simulink model "simulink_model"  (R2020b)
settings: Solver=VariableStepAuto  StartTime=0.0  StopTime=10  MaxStep=1e-3  RelTol=1e-5  AbsTol=1e-5
InitFcn:
  | % Init Walking SLIP
  | m = 80;
  | g = 9.81;
  | kk = 10000;
  | l0 = 1;
  | aTD = 68*pi/180;
  | E = 810;
  | x0 = 0;
  | y0 = 0.97;
  | dx0 = 1.05;
  | dy0 = 0;
  | yTD = l0*sin(aTD);
settings Model: Creator=ASUS  LastModifiedBy=edizferit
settings DataIOCC: ReturnWorkspaceOutputs=off

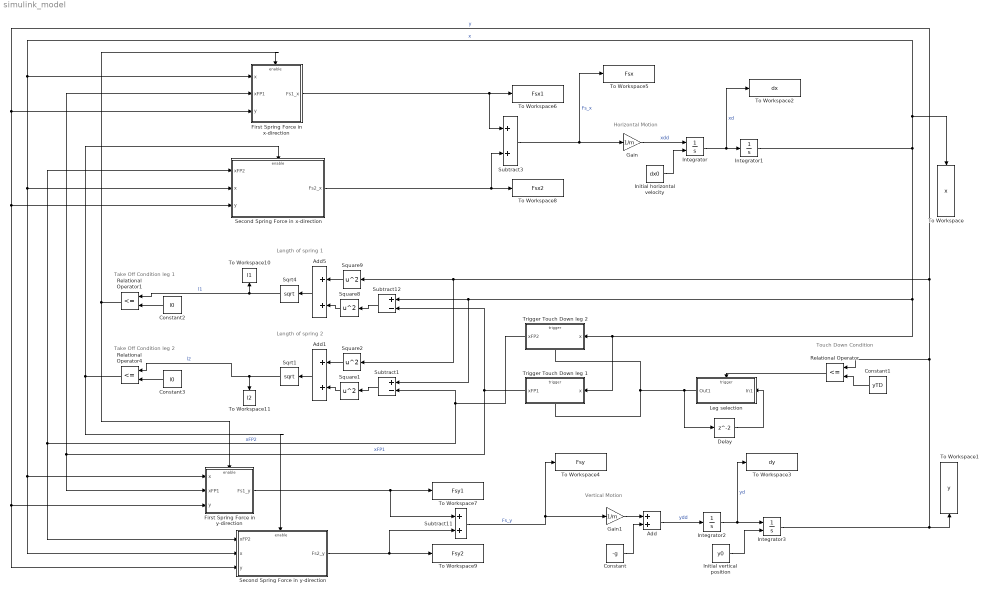
== system simulink_model ==
  note: Touch Down Condition
  note: Take Off Condition leg 1
  note: Vertical Motion
  note: Horizontal Motion
  note: Length of spring 1
  note: Length of spring 2
  note: Take Off Condition leg 2
  Add : Sum
  Add1 : Sum
  Add5 : Sum
  Constant : Constant  Value=-g
  Constant1 : Constant  Value=yTD
  Constant2 : Constant  Value=l0
  Constant3 : Constant  Value=l0
  Delay : Delay
  First Spring Force in x-direction : Subsystem
  First Spring Force in y-direction : Subsystem
  Gain : Gain  Gain=1/m
  Gain1 : Gain  Gain=1/m
  Initial horizontal velocity : Constant  InitFcn=|  Value=dx0
      | %% Init Running SLIP
      | m = 80;
      | g = 9.81;
      | k = 10;
      | l0 = 1;
      | aTD = 68*pi/180;
      | E = 810;
      | x0 = 0;
      | y0 = 0.97;
      | dx0 = 1.05;
      | dy0 = 0;
      | yTD = l0*sin(aTD);
  Initial vertical position : Constant  Value=y0
  Integrator : Integrator  InitialConditionSource=external
  Integrator1 : Integrator
  Integrator2 : Integrator
  Integrator3 : Integrator  InitialConditionSource=external
  "Leg selection " : Subsystem  TreatAsAtomicUnit=on
  Relational Operator : RelationalOperator  Operator=<=  OutDataTypeStr=boolean  RndMeth=Simplest
  Relational Operator1 : RelationalOperator  Operator=<=  OutDataTypeStr=boolean  RndMeth=Simplest
  Relational Operator4 : RelationalOperator  Operator=<=  OutDataTypeStr=boolean  RndMeth=Simplest
  Second Spring Force in x-direction : Subsystem
  Second Spring Force in y-direction : Subsystem
  Sqrt1 : Sqrt  SaturateOnIntegerOverflow=on
  Sqrt4 : Sqrt  SaturateOnIntegerOverflow=on
  Square{1..2,8..9} (4 alike) : Math  Operator=square  SaturateOnIntegerOverflow=on
  Subtract1 : Sum  Inputs=+-
  Subtract11 : Sum
  Subtract12 : Sum  Inputs=+-
  Subtract3 : Sum
  To Workspace : ToWorkspace  VariableName=x  SaveFormat=Timeseries  SampleTime=-1
  To Workspace1 : ToWorkspace  VariableName=y  SaveFormat=Timeseries  SampleTime=-1
  To Workspace10 : ToWorkspace  VariableName=l1  SaveFormat=Timeseries  SampleTime=-1
  To Workspace11 : ToWorkspace  VariableName=l2  SaveFormat=Timeseries  SampleTime=-1
  To Workspace2 : ToWorkspace  VariableName=dx  SaveFormat=Timeseries  SampleTime=-1
  To Workspace3 : ToWorkspace  VariableName=dy  SaveFormat=Timeseries  SampleTime=-1
  To Workspace4 : ToWorkspace  VariableName=Fsy  SaveFormat=Timeseries  SampleTime=-1
  To Workspace5 : ToWorkspace  VariableName=Fsx  SaveFormat=Timeseries  SampleTime=-1
  To Workspace6 : ToWorkspace  VariableName=Fsx1  SaveFormat=Timeseries  SampleTime=-1
  To Workspace7 : ToWorkspace  VariableName=Fsy1  SaveFormat=Timeseries  SampleTime=-1
  To Workspace8 : ToWorkspace  VariableName=Fsx2  SaveFormat=Timeseries  SampleTime=-1
  To Workspace9 : ToWorkspace  VariableName=Fsy2  SaveFormat=Timeseries  SampleTime=-1
  Trigger Touch Down leg 1 : Subsystem  TreatAsAtomicUnit=on
  Trigger Touch Down leg 2 : Subsystem  TreatAsAtomicUnit=on
  wires:
  Gain/1 -> Integrator/1  "xdd"
  Integrator/1 -> To Workspace2/1, Integrator1/1  "xd"
  Initial horizontal velocity/1 -> Integrator/2
  Initial vertical position/1 -> Integrator3/2
  Add/1 -> Integrator2/1  "ydd"
  Gain1/1 -> Add/1
  Constant/1 -> Add/2
  Constant1/1 -> Relational Operator/2
  Constant2/1 -> Relational Operator1/2
  Sqrt4/1 -> Relational Operator1/1, To Workspace10/1  "l1"
  Integrator3/1 -> Second Spring Force in y-direction/3(y), First Spring Force in y-direction/3(y), Second Spring Force in x-direction/3(y), First Spring Force in x-direction/3(y), Square2/1, Square9/1, Relational Operator/1, To Workspace1/1  "y"
  Subtract12/1 -> Square8/1
  Add5/1 -> Sqrt4/1
  Square9/1 -> Add5/1
  Square8/1 -> Add5/2
  Trigger Touch Down leg 2/1(xFP2) -> Second Spring Force in x-direction/1(xFP2), Second Spring Force in y-direction/1(xFP2), Subtract1/2  "xFP2"
  Trigger Touch Down leg 1/1(xFP1) -> First Spring Force in x-direction/2(xFP1), First Spring Force in y-direction/2(xFP1), Subtract12/2  "xFP1"
  Second Spring Force in y-direction/1(Fs2_y) -> To Workspace9/1, Subtract11/2
  First Spring Force in y-direction/1(Fs1_y) -> To Workspace7/1, Subtract11/1
  First Spring Force in x-direction/1(Fs1_x) -> To Workspace6/1, Subtract3/1
  Second Spring Force in x-direction/1(Fs2_x) -> To Workspace8/1, Subtract3/2
  Relational Operator/1 -> "Leg selection "/Trigger
  "Leg selection "/1(Out1) -> Delay/1, Trigger Touch Down leg 2/Trigger, Trigger Touch Down leg 1/Trigger
  Delay/1 -> "Leg selection "/1(In1)
  Square1/1 -> Add1/2
  Square2/1 -> Add1/1
  Add1/1 -> Sqrt1/1
  Subtract1/1 -> Square1/1
  Constant3/1 -> Relational Operator4/2
  Sqrt1/1 -> Relational Operator4/1, To Workspace11/1  "l2"
  Relational Operator1/1 -> First Spring Force in x-direction/Enable, First Spring Force in y-direction/Enable
  Relational Operator4/1 -> Second Spring Force in x-direction/Enable, Second Spring Force in y-direction/Enable
  Integrator2/1 -> To Workspace3/1, Integrator3/1  "yd"
  Subtract11/1 -> To Workspace4/1, Gain1/1  "Fs_y"
  Integrator1/1 -> To Workspace/1, Second Spring Force in y-direction/2(x), First Spring Force in y-direction/1(x), Second Spring Force in x-direction/2(x), First Spring Force in x-direction/1(x), Trigger Touch Down leg 1/1(x), Trigger Touch Down leg 2/1(x), Subtract12/1, Subtract1/1  "x"
  Subtract3/1 -> To Workspace5/1, Gain/1  "Fs_x"

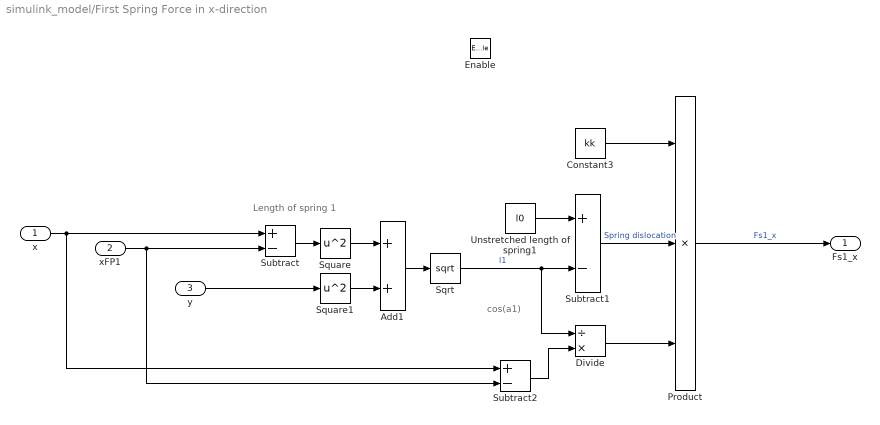
== system simulink_model/First Spring Force in x-direction ==
  note: cos(a1)
  note: Length of spring 1
  x : Inport
  xFP1 : Inport  Port=2
  y : Inport  Port=3
  Enable : EnablePort  StatesWhenEnabling=reset
  Add1 : Sum
  Constant3 : Constant  Value=kk
  Divide : Product  Inputs=/*
  Product : Product  Inputs=3
  Sqrt : Sqrt  SaturateOnIntegerOverflow=on
  Square : Math  Operator=square  SaturateOnIntegerOverflow=on
  Square1 : Math  Operator=square  SaturateOnIntegerOverflow=on
  Subtract : Sum  Inputs=+-
  Subtract1 : Sum  Inputs=+-
  Subtract2 : Sum  Inputs=+-
  Unstretched length of spring1 : Constant  Value=l0
  Fs1_x : Outport
  wires:
  Sqrt/1 -> Divide/1, Subtract1/2  "l1"
  Add1/1 -> Sqrt/1
  Subtract/1 -> Square/1
  Constant3/1 -> Product/1
  Subtract1/1 -> Product/2  "Spring dislocation"
  Unstretched length of spring1/1 -> Subtract1/1
  Square1/1 -> Add1/2
  Divide/1 -> Product/3
  Subtract2/1 -> Divide/2
  Square/1 -> Add1/1
  xFP1/1 -> Subtract2/2, Subtract/2
  x/1 -> Subtract2/1, Subtract/1
  Product/1 -> Fs1_x/1  "Fs1_x"
  y/1 -> Square1/1

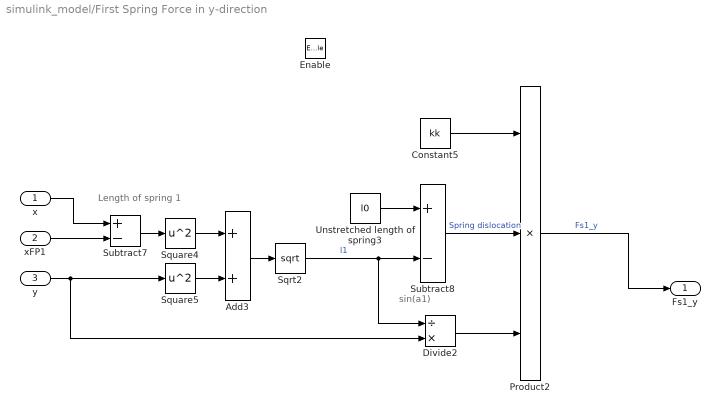
== system simulink_model/First Spring Force in y-direction ==
  note: sin(a1)
  note: Length of spring 1
  x : Inport
  xFP1 : Inport  Port=2
  y : Inport  Port=3
  Enable : EnablePort  StatesWhenEnabling=reset
  Add3 : Sum
  Constant5 : Constant  Value=kk
  Divide2 : Product  Inputs=/*
  Product2 : Product  Inputs=3
  Sqrt2 : Sqrt  SaturateOnIntegerOverflow=on
  Square4 : Math  Operator=square  SaturateOnIntegerOverflow=on
  Square5 : Math  Operator=square  SaturateOnIntegerOverflow=on
  Subtract7 : Sum  Inputs=+-
  Subtract8 : Sum  Inputs=+-
  Unstretched length of spring3 : Constant  Value=l0
  Fs1_y : Outport
  wires:
  Subtract8/1 -> Product2/2  "Spring dislocation"
  Divide2/1 -> Product2/3
  Unstretched length of spring3/1 -> Subtract8/1
  Subtract7/1 -> Square4/1
  Add3/1 -> Sqrt2/1
  Square5/1 -> Add3/2
  Sqrt2/1 -> Divide2/1, Subtract8/2  "l1"
  Square4/1 -> Add3/1
  x/1 -> Subtract7/1
  Constant5/1 -> Product2/1
  y/1 -> Divide2/2, Square5/1
  xFP1/1 -> Subtract7/2
  Product2/1 -> Fs1_y/1  "Fs1_y"

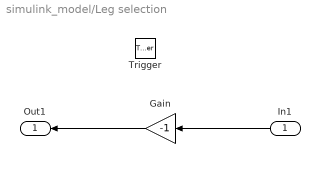
== system simulink_model/Leg selection  ==
  In1 : Inport
  Trigger : TriggerPort  VariantControl=Variant
  Gain : Gain  Gain=-1
  Out1 : Outport  InitialOutput=[1]
  wires:
  In1/1 -> Gain/1
  Gain/1 -> Out1/1

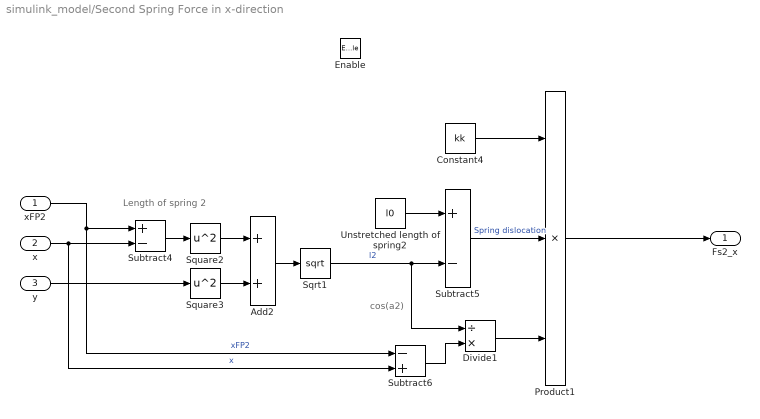
== system simulink_model/Second Spring Force in x-direction ==
  note: cos(a2)
  note: Length of spring 2
  xFP2 : Inport
  x : Inport  Port=2
  y : Inport  Port=3
  Enable : EnablePort  StatesWhenEnabling=reset
  Add2 : Sum
  Constant4 : Constant  Value=kk
  Divide1 : Product  Inputs=/*
  Product1 : Product  Inputs=3
  Sqrt1 : Sqrt  SaturateOnIntegerOverflow=on
  Square2 : Math  Operator=square  SaturateOnIntegerOverflow=on
  Square3 : Math  Operator=square  SaturateOnIntegerOverflow=on
  Subtract4 : Sum  Inputs=+-
  Subtract5 : Sum  Inputs=+-
  Subtract6 : Sum  Inputs=-+
  Unstretched length of spring2 : Constant  Value=l0
  Fs2_x : Outport  OutputWhenDisabled=reset  InitialOutput=[0]
  wires:
  Subtract4/1 -> Square2/1
  Sqrt1/1 -> Divide1/1, Subtract5/2  "l2"
  Subtract6/1 -> Divide1/2
  Square3/1 -> Add2/2
  Square2/1 -> Add2/1
  xFP2/1 -> Subtract6/1, Subtract4/1  "xFP2"
  x/1 -> Subtract6/2, Subtract4/2  "x"
  Constant4/1 -> Product1/1
  Divide1/1 -> Product1/3
  Unstretched length of spring2/1 -> Subtract5/1
  Add2/1 -> Sqrt1/1
  Subtract5/1 -> Product1/2  "Spring dislocation"
  Product1/1 -> Fs2_x/1
  y/1 -> Square3/1

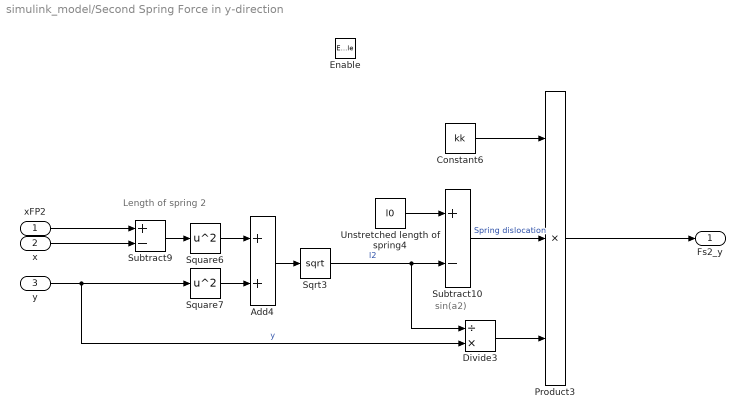
== system simulink_model/Second Spring Force in y-direction ==
  note: sin(a2)
  note: Length of spring 2
  xFP2 : Inport
  x : Inport  Port=2
  y : Inport  Port=3
  Enable : EnablePort  StatesWhenEnabling=reset
  Add4 : Sum
  Constant6 : Constant  Value=kk
  Divide3 : Product  Inputs=/*
  Product3 : Product  Inputs=3
  Sqrt3 : Sqrt  SaturateOnIntegerOverflow=on
  Square6 : Math  Operator=square  SaturateOnIntegerOverflow=on
  Square7 : Math  Operator=square  SaturateOnIntegerOverflow=on
  Subtract10 : Sum  Inputs=+-
  Subtract9 : Sum  Inputs=+-
  Unstretched length of spring4 : Constant  Value=l0
  Fs2_y : Outport  OutputWhenDisabled=reset  InitialOutput=[0]
  wires:
  Unstretched length of spring4/1 -> Subtract10/1
  Constant6/1 -> Product3/1
  Add4/1 -> Sqrt3/1
  Subtract9/1 -> Square6/1
  Square7/1 -> Add4/2
  Square6/1 -> Add4/1
  Sqrt3/1 -> Divide3/1, Subtract10/2  "l2"
  Divide3/1 -> Product3/3
  Subtract10/1 -> Product3/2  "Spring dislocation"
  x/1 -> Subtract9/2
  y/1 -> Divide3/2, Square7/1  "y"
  xFP2/1 -> Subtract9/1
  Product3/1 -> Fs2_y/1

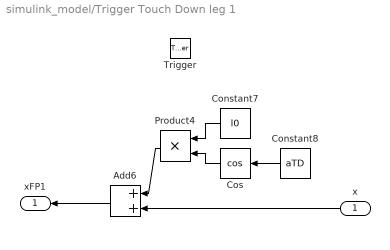
== system simulink_model/Trigger Touch Down leg 1 ==
  x : Inport
  Trigger : TriggerPort  VariantControl=Variant
  Add6 : Sum
  Constant7 : Constant  Value=l0
  Constant8 : Constant  Value=aTD
  Cos : Trigonometry  Operator=cos
  Product4 : Product
  xFP1 : Outport  InitialOutput=[0]
  wires:
  x/1 -> Add6/2
  Constant8/1 -> Cos/1
  Add6/1 -> xFP1/1
  Constant7/1 -> Product4/1
  Product4/1 -> Add6/1
  Cos/1 -> Product4/2

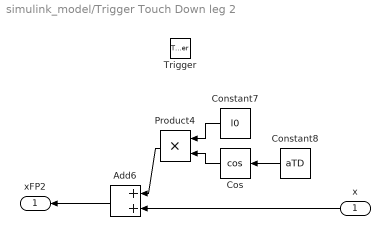
== system simulink_model/Trigger Touch Down leg 2 ==
  x : Inport
  Trigger : TriggerPort  TriggerType=falling  VariantControl=Variant
  Add6 : Sum
  Constant7 : Constant  Value=l0
  Constant8 : Constant  Value=aTD
  Cos : Trigonometry  Operator=cos
  Product4 : Product
  xFP2 : Outport  InitialOutput=[-1]
  wires:
  Cos/1 -> Product4/2
  Product4/1 -> Add6/1
  Constant7/1 -> Product4/1
  Add6/1 -> xFP2/1
  Constant8/1 -> Cos/1
  x/1 -> Add6/2
